simulink model "Dynamic_model_2021b"  (R2021b)
settings: Solver=VariableStepAuto  StartTime=0.0  StopTime=10.0  RelTol=1e-3
values from neighbouring files (symbols this model uses):
  param = struct()    [parameters.m]
libraries: dspmtrx3 x3, sharedtransform x2, matrix_library x1
settings Model: Creator=volko  LastModifiedBy=volko

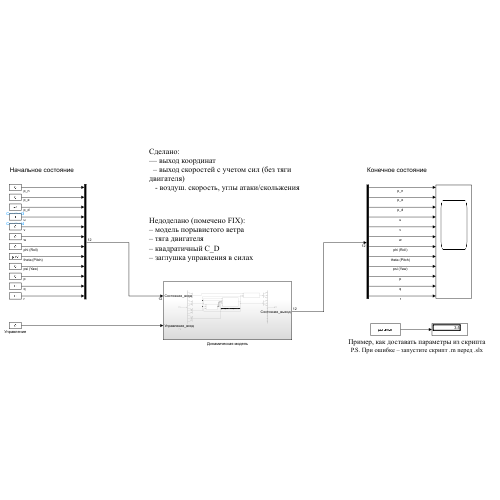
[thumbnail: Simulink's stored preview of the top-level diagram]
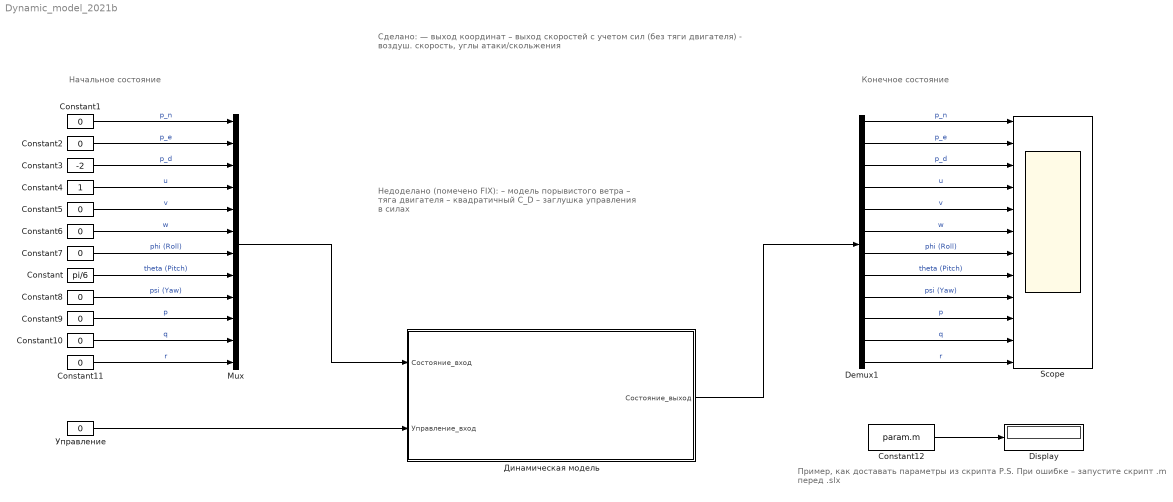
== system Dynamic_model_2021b ==
  note: Сделано:
      | — выход координат
      | – выход скоростей с учетом сил (без тяги двигателя)
      | - воздуш. скорость, углы атаки/скольжения
  note: Пример, как доставать параметры из скрипта
      | P.S. При ошибке – запустите скрипт .m перед .slx
  note: Начальное состояние
  note: Недоделано (помечено FIX):
      | – модель порывистого ветра
      | – тяга двигателя
      | – квадратичный C_D
      | – заглушка управления в силах
  note: Конечное состояние
  Constant : Constant  Value=pi/6
  Constant{1..2,5..11} (9 alike) : Constant  Value=0
  Constant12 : Constant  Value=param.m
  Constant3 : Constant  Value=-2
  Constant4 : Constant
  Demux1 : Demux  Outputs=12
  Display : Display
  Mux : Mux  Inputs=12
  Scope : Scope  NumInputPorts=12
  Динамическая модель : Subsystem
  Управление : Constant  Value=0
  wires:
  Constant7/1 -> Mux/7  "phi (Roll)"
  Demux1/11 -> Scope/11  "q"
  Demux1/1 -> Scope/1  "p_n"
  Mux/1 -> Динамическая модель/1(Состояние_вход)
  Demux1/9 -> Scope/9  "psi (Yaw)"
  Constant2/1 -> Mux/2  "p_e"
  Demux1/3 -> Scope/3  "p_d"
  Constant12/1 -> Display/1
  Demux1/10 -> Scope/10  "p"
  Demux1/12 -> Scope/12  "r"
  Constant10/1 -> Mux/11  "q"
  Управление/1 -> Динамическая модель/2(Управление_вход)
  Demux1/7 -> Scope/7  "phi (Roll)"
  Constant/1 -> Mux/8  "theta (Pitch)"
  Constant3/1 -> Mux/3  "p_d"
  Demux1/5 -> Scope/5  "v"
  Constant5/1 -> Mux/5  "v"
  Demux1/2 -> Scope/2  "p_e"
  Динамическая модель/1(Состояние_выход) -> Demux1/1
  Demux1/6 -> Scope/6  "w"
  Constant11/1 -> Mux/12  "r"
  Constant1/1 -> Mux/1  "p_n"
  Demux1/4 -> Scope/4  "u"
  Constant4/1 -> Mux/4  "u"
  Constant8/1 -> Mux/9  "psi (Yaw)"
  Constant9/1 -> Mux/10  "p"
  Demux1/8 -> Scope/8  "theta (Pitch)"
  Constant6/1 -> Mux/6  "w"

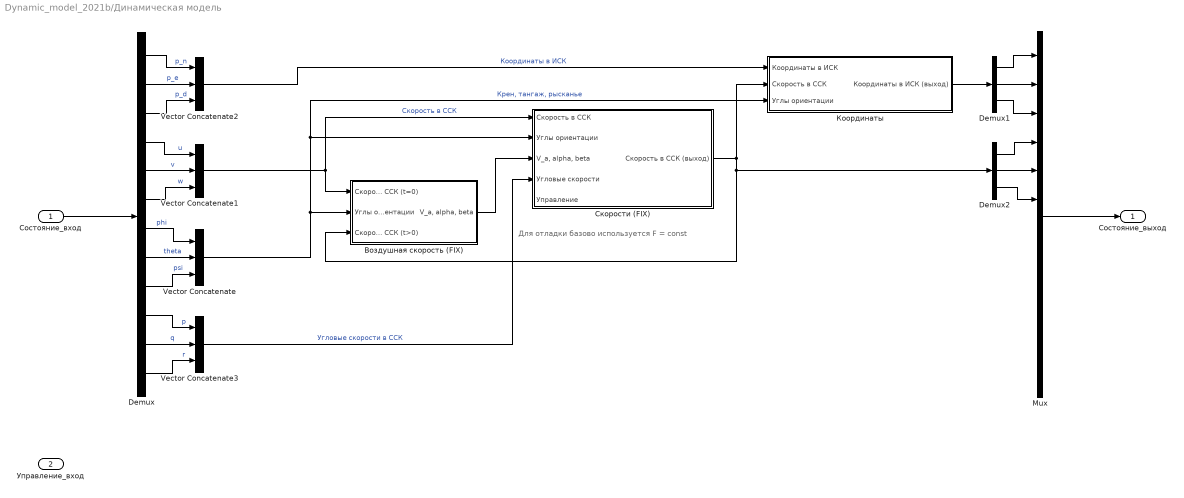
== system Dynamic_model_2021b/Динамическая модель ==
  note: Для отладки базово используется F = const
  Состояние_вход : Inport
  Управление_вход : Inport  Port=2
  Demux : Demux  Outputs=12
  Demux1 : Demux  Outputs=3
  Demux2 : Demux  Outputs=3
  Mux : Mux  Inputs=12
  Vector Concatenate{,1..3} (4 alike) : Concatenate  NumInputs=3
  Воздушная скорость (FIX) : Subsystem
  Координаты : Subsystem
  Скорости (FIX) : Subsystem
  Состояние_выход : Outport
  wires:
  Состояние_вход/1 -> Demux/1
  Demux/1 -> Vector Concatenate2/1  "p_n"
  Demux/2 -> Vector Concatenate2/2  "p_e"
  Demux/3 -> Vector Concatenate2/3  "p_d"
  Demux/4 -> Vector Concatenate1/1  "u"
  Demux/5 -> Vector Concatenate1/2  "v"
  Demux/6 -> Vector Concatenate1/3  "w"
  Demux/7 -> Vector Concatenate/1  "phi"
  Demux/8 -> Vector Concatenate/2  "theta"
  Demux/9 -> Vector Concatenate/3  "psi"
  Demux/10 -> Vector Concatenate3/1  "p"
  Demux/11 -> Vector Concatenate3/2  "q"
  Demux/12 -> Vector Concatenate3/3  "r"
  Vector Concatenate2/1 -> Координаты/1(Координаты в ИСК)  "Координаты в ИСК"
  Vector Concatenate1/1 -> Воздушная скорость (FIX)/1(Скорость в ССК (t=0)), Скорости (FIX)/1(Скорость в ССК)  "Скорость в ССК"
  Vector Concatenate/1 -> Воздушная скорость (FIX)/2(Углы ориентации), Скорости (FIX)/2(Углы ориентации), Координаты/3(Углы ориентации)  "Крен, тангаж, рысканье"
  Координаты/1(Координаты в ИСК (выход)) -> Demux1/1
  Vector Concatenate3/1 -> Скорости (FIX)/4(Угловые скорости)  "Угловые скорости в ССК"
  Mux/1 -> Состояние_выход/1
  Demux1/1 -> Mux/1
  Demux1/2 -> Mux/2
  Demux1/3 -> Mux/3
  Demux2/2 -> Mux/5
  Demux2/1 -> Mux/4
  Demux2/3 -> Mux/6
  Воздушная скорость (FIX)/1("V_a, alpha, beta") -> Скорости (FIX)/3("V_a, alpha, beta")
  Скорости (FIX)/1(Скорость в ССК (выход)) -> Координаты/2(Скорость в ССК), Воздушная скорость (FIX)/3(Скорость в ССК (t>0)), Demux2/1

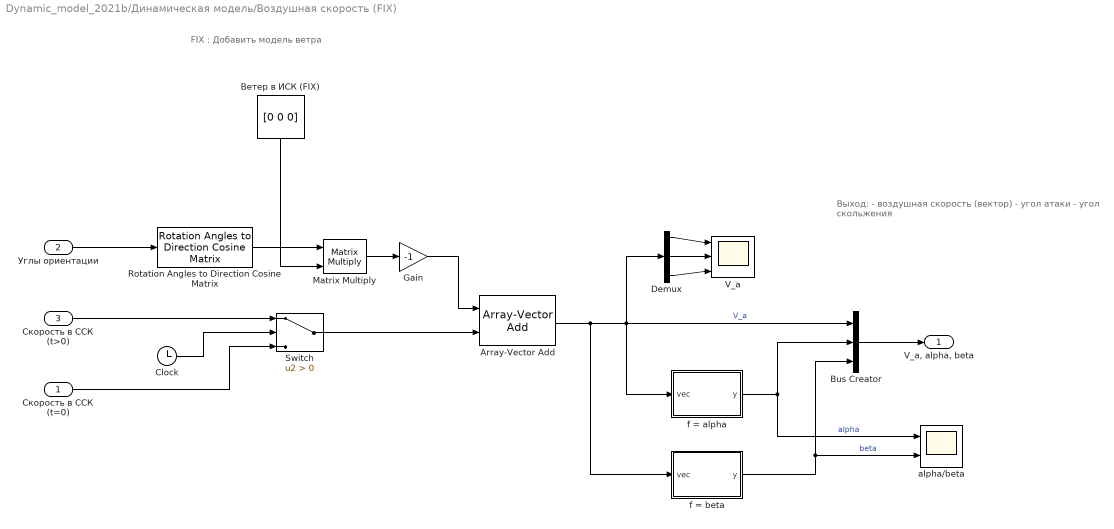
== system Dynamic_model_2021b/Динамическая модель/Воздушная скорость (FIX) ==
  note: Выход:
      | - воздушная скорость (вектор)
      | - угол атаки
      | - угол скольжения
  note: FIX : Добавить модель ветра
  Скорость в ССК (t=0) : Inport
  Углы ориентации : Inport  Port=2
  Скорость в ССК (t>0) : Inport  Port=3
  Array-Vector Add : dspmtrx3/Array-Vector Add  Dimension=1  V_Source=Input port  V_VectFromMask=[0.5 0.25]  prodOutputSignedness=Auto  roundingMode=Floor  overflowMode=off  firstCoeffSignedness=Auto  firstCoeffDataTypeStr=Inherit: Same word length as input  firstCoeffMin=[]  firstCoeffMax=[]  firstCoeffLastDataTypeStr=Inherit: Same word length as input  accumSignedness=Auto  outputSignedness=Auto  outputDataTypeStr=Inherit: Same as accumulator  outputMin=[]  outputMax=[]  outputLastDataTypeStr=Inherit: Same as accumulator
      settings: SourceProductBaseCode=DS
  Bus Creator : BusCreator  Inputs=3
  Clock : Clock
  Demux : Demux  Outputs=3
  Gain : Gain  Gain=-1
  Matrix Multiply : Product  Multiplication=Matrix(*)
  Rotation Angles to Direction Cosine Matrix : sharedtransform/Rotation Angles to Direction Cosine Matrix  rotationOrder=XYZ  aMode=aMode
      settings: SourceProductBaseCode=AE,PW,DR,MT,UV,VE
  Switch : Switch  Criteria=u2 > Threshold
  V_a : Scope  NumInputPorts=3
  alpha/beta : Scope  NumInputPorts=2
  f = alpha : MATLAB Function  TreatAsAtomicUnit=on
  f = beta : MATLAB Function  TreatAsAtomicUnit=on
  Ветер в ИСК (FIX) : Constant  Value=[0 0 0]
  "V_a, alpha, beta" : Outport
  wires:
  Скорость в ССК (t=0)/1 -> Switch/3
  Ветер в ИСК (FIX)/1 -> Matrix Multiply/2
  Array-Vector Add/1 -> Bus Creator/1, Demux/1, f = alpha/1(vec), f = beta/1(vec)  "V_a"
  Rotation Angles to Direction Cosine Matrix/1 -> Matrix Multiply/1
  Углы ориентации/1 -> Rotation Angles to Direction Cosine Matrix/1
  Matrix Multiply/1 -> Gain/1
  f = beta/1(y) -> Bus Creator/3, alpha/beta/2  "beta"
  f = alpha/1(y) -> alpha/beta/1, Bus Creator/2  "alpha"
  Bus Creator/1 -> "V_a, alpha, beta"/1
  Gain/1 -> Array-Vector Add/1
  Demux/1 -> V_a/1
  Demux/2 -> V_a/2
  Demux/3 -> V_a/3
  Clock/1 -> Switch/2
  Скорость в ССК (t>0)/1 -> Switch/1
  Switch/1 -> Array-Vector Add/2

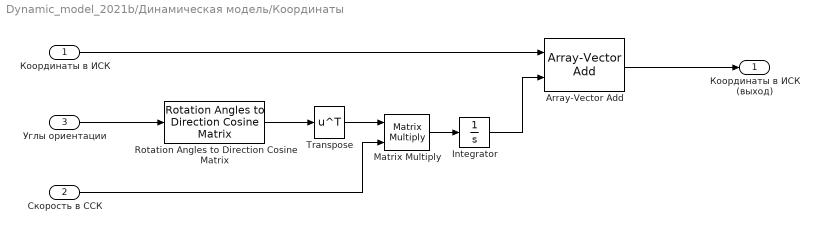
== system Dynamic_model_2021b/Динамическая модель/Координаты ==
  Координаты в ИСК : Inport
  Скорость в ССК : Inport  Port=2
  Углы ориентации : Inport  Port=3
  Array-Vector Add : dspmtrx3/Array-Vector Add  Dimension=1  V_Source=Input port  V_VectFromMask=[0.5 0.25]  prodOutputSignedness=Auto  roundingMode=Floor  overflowMode=off  firstCoeffSignedness=Auto  firstCoeffDataTypeStr=Inherit: Same word length as input  firstCoeffMin=[]  firstCoeffMax=[]  firstCoeffLastDataTypeStr=Inherit: Same word length as input  accumSignedness=Auto  outputSignedness=Auto  outputDataTypeStr=Inherit: Same as accumulator  outputMin=[]  outputMax=[]  outputLastDataTypeStr=Inherit: Same as accumulator
      settings: SourceProductBaseCode=DS
  Integrator : Integrator
  Matrix Multiply : Product  Multiplication=Matrix(*)
  Rotation Angles to Direction Cosine Matrix : sharedtransform/Rotation Angles to Direction Cosine Matrix  rotationOrder=XYZ  aMode=aMode
      settings: SourceProductBaseCode=AE,PW,DR,MT,UV,VE
  Transpose : Math  Operator=transpose  SaturateOnIntegerOverflow=on
  Координаты в ИСК (выход) : Outport
  wires:
  Скорость в ССК/1 -> Matrix Multiply/2
  Integrator/1 -> Array-Vector Add/2
  Rotation Angles to Direction Cosine Matrix/1 -> Transpose/1
  Transpose/1 -> Matrix Multiply/1
  Углы ориентации/1 -> Rotation Angles to Direction Cosine Matrix/1
  Array-Vector Add/1 -> Координаты в ИСК (выход)/1
  Координаты в ИСК/1 -> Array-Vector Add/1
  Matrix Multiply/1 -> Integrator/1

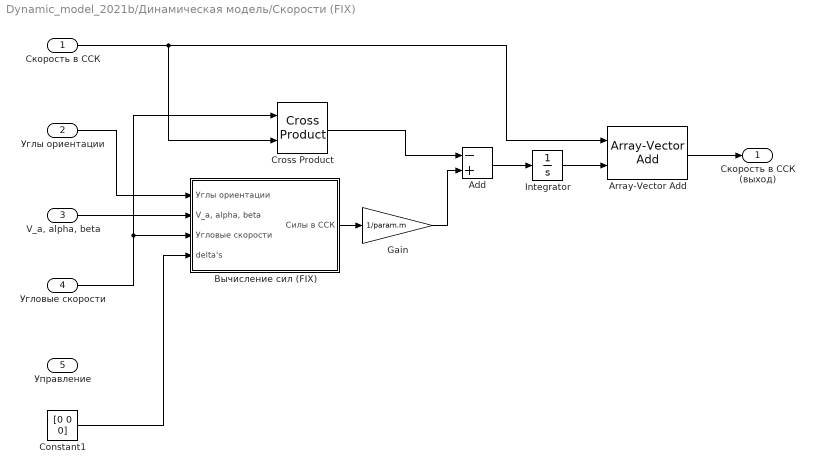
== system Dynamic_model_2021b/Динамическая модель/Скорости (FIX) ==
  Скорость в ССК : Inport
  Углы ориентации : Inport  Port=2
  "V_a, alpha, beta" : Inport  Port=3
  Угловые скорости : Inport  Port=4
  Управление : Inport  Port=5
  Add : Sum  Inputs=-+
  Array-Vector Add : dspmtrx3/Array-Vector Add  Dimension=1  V_Source=Input port  V_VectFromMask=[0.5 0.25]  prodOutputSignedness=Auto  roundingMode=Floor  overflowMode=off  firstCoeffSignedness=Auto  firstCoeffDataTypeStr=Inherit: Same word length as input  firstCoeffMin=[]  firstCoeffMax=[]  firstCoeffLastDataTypeStr=Inherit: Same word length as input  accumSignedness=Auto  outputSignedness=Auto  outputDataTypeStr=Inherit: Same as accumulator  outputMin=[]  outputMax=[]  outputLastDataTypeStr=Inherit: Same as accumulator
      settings: SourceProductBaseCode=DS
  Constant1 : Constant  Value=[0 0 0]
  Cross Product : matrix_library/Cross Product
      settings: SourceProductBaseCode=SL
  Gain : Gain  Gain=1/param.m
  Integrator : Integrator
  Вычисление сил (FIX) : Subsystem
  Скорость в ССК (выход) : Outport
  wires:
  Угловые скорости/1 -> Cross Product/1, Вычисление сил (FIX)/3(Угловые скорости)
  Скорость в ССК/1 -> Array-Vector Add/1, Cross Product/2
  Вычисление сил (FIX)/1(Силы в ССК) -> Gain/1
  Cross Product/1 -> Add/1
  Gain/1 -> Add/2
  Integrator/1 -> Array-Vector Add/2
  Add/1 -> Integrator/1
  Array-Vector Add/1 -> Скорость в ССК (выход)/1
  Углы ориентации/1 -> Вычисление сил (FIX)/1(Углы ориентации)
  "V_a, alpha, beta"/1 -> Вычисление сил (FIX)/2("V_a, alpha, beta")
  Constant1/1 -> Вычисление сил (FIX)/4(delta's)

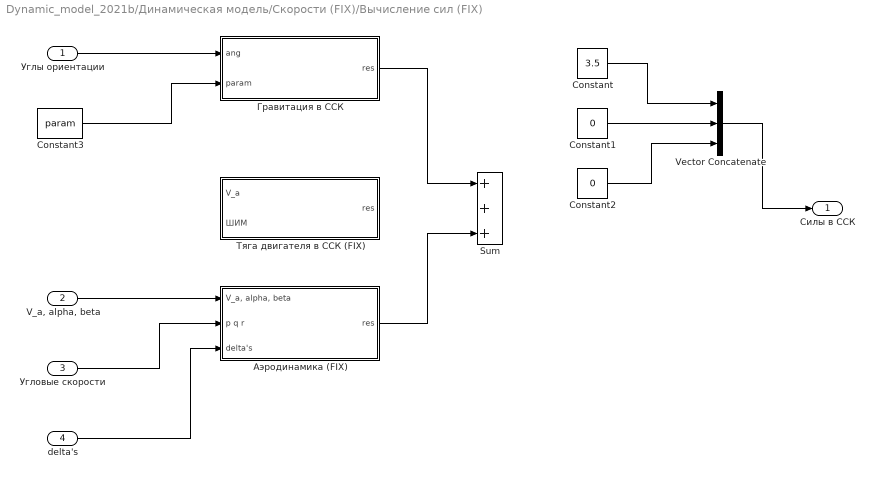
== system Dynamic_model_2021b/Динамическая модель/Скорости (FIX)/Вычисление сил (FIX) ==
  Углы ориентации : Inport
  "V_a, alpha, beta" : Inport  Port=2
  Угловые скорости : Inport  Port=3
  delta's : Inport  Port=4
  Constant : Constant  Value=3.5
  Constant1 : Constant  Value=0
  Constant2 : Constant  Value=0
  Constant3 : Constant  Value=param  OutDataTypeStr=Bus: slBus1
  Sum : Sum  Inputs=+++
  Vector Concatenate : Concatenate  NumInputs=3
  Аэродинамика (FIX) : Subsystem
  Гравитация в ССК : MATLAB Function  TreatAsAtomicUnit=on
  Тяга двигателя в ССК (FIX) : Subsystem
  Силы в ССК : Outport
  wires:
  Constant/1 -> Vector Concatenate/1
  Constant1/1 -> Vector Concatenate/2
  Constant2/1 -> Vector Concatenate/3
  Углы ориентации/1 -> Гравитация в ССК/1(ang)
  Constant3/1 -> Гравитация в ССК/2(param)
  "V_a, alpha, beta"/1 -> Аэродинамика (FIX)/1("V_a, alpha, beta")
  Угловые скорости/1 -> Аэродинамика (FIX)/2(p q r)
  delta's/1 -> Аэродинамика (FIX)/3(delta's)
  Аэродинамика (FIX)/1(res) -> Sum/3
  Гравитация в ССК/1(res) -> Sum/1
  Vector Concatenate/1 -> Силы в ССК/1

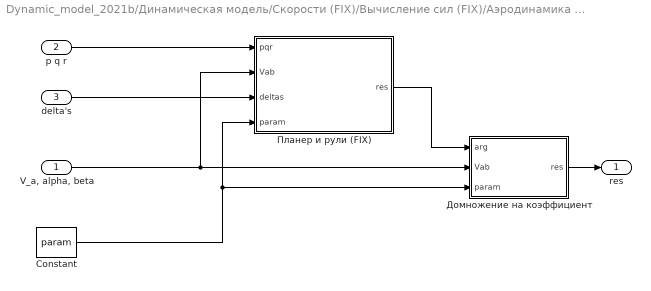
== system Dynamic_model_2021b/Динамическая модель/Скорости (FIX)/Вычисление сил (FIX)/Аэродинамика (FIX) ==
  "V_a, alpha, beta" : Inport
  p q r : Inport  Port=2
  delta's : Inport  Port=3
  Constant : Constant  Value=param  OutDataTypeStr=Bus: slBus1
  Домножение на коэффициент : MATLAB Function  TreatAsAtomicUnit=on
  Планер и рули (FIX) : MATLAB Function  TreatAsAtomicUnit=on
  res : Outport
  wires:
  Домножение на коэффициент/1(res) -> res/1
  Constant/1 -> Планер и рули (FIX)/4(param), Домножение на коэффициент/3(param)
  "V_a, alpha, beta"/1 -> Планер и рули (FIX)/2(Vab), Домножение на коэффициент/2(Vab)
  p q r/1 -> Планер и рули (FIX)/1(pqr)
  Планер и рули (FIX)/1(res) -> Домножение на коэффициент/1(arg)
  delta's/1 -> Планер и рули (FIX)/3(deltas)

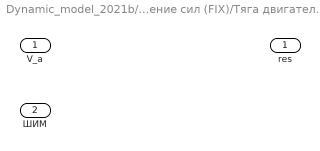
== system Dynamic_model_2021b/Динамическая модель/Скорости (FIX)/Вычисление сил (FIX)/Тяга двигателя в ССК (FIX) ==
  V_a : Inport
  ШИМ : Inport  Port=2
  res : Outport

== matlab function Dynamic_model_2021b/Динамическая модель/Воздушная скорость (FIX)/f = beta ==
  data: vec input; y output
function y = fcn(vec)

y = asin( vec(2) / norm(vec) );

== matlab function Dynamic_model_2021b/Динамическая модель/Воздушная скорость (FIX)/f = alpha ==
  data: vec input; y output
function y = fcn(vec)

y = atan( vec(3) / vec(1) );

== matlab function Dynamic_model_2021b/Динамическая модель/Скорости (FIX)/Вычисление сил (FIX)/Гравитация в ССК ==
  data: ang input; res output; param input
function res = fcn(ang, param)
phi = ang(1);
theta = ang(2);
x = -param.m * param.g * sin(theta);
y = param.m * param.g * cos(theta) * sin(phi);
z = param.m * param.g * cos(theta) * cos(phi);
res = [x y z];

== matlab function Dynamic_model_2021b/Динамическая модель/Скорости (FIX)/Вычисление сил (FIX)/Аэродинамика (FIX)/Домножение на коэффициент ==
  data: arg input; res output; Vab input; param input
function res = fcn(arg, Vab, param)
V_a = Vab(1:3);
res = arg * 0.5 * param.rho * norm(V_a)^2 * param.S;

== matlab function Dynamic_model_2021b/Динамическая модель/Скорости (FIX)/Вычисление сил (FIX)/Аэродинамика (FIX)/Планер и рули (FIX) ==
  data: pqr input; res output; Vab input; deltas input; param input
function res = fcn(pqr, Vab, deltas, param)
% pqr = угловые скорости в ССК
% Vab = воздушная скорость, угол атаки и скольжения
% deltas = отклонения рулей
vV_a = Vab(1:3);
V_a = norm(Vab(1:3));
a = Vab(4);
beta = Vab(5);
p = pqr(1);
q = pqr(2);
r = pqr(3);
delta_a = deltas(1);
delta_e = deltas(2);
delta_r = deltas(3);

%C_D упрощен до линейного !!!!!!!!!!!!!!!!!!!!!!!!!
C_D = param.C_D0 + param.C_Da * a + param.C_Dde * delta_e + param.C_Dq * param.c * q / (2*V_a);
C_L = param.C_L0 + param.C_La * a + param.C_Lde * delta_e + param.C_Lq * param.c * q / (2*V_a);

C = ([cos(a) -sin(a); sin(a) cos(a) ] * [-C_D; -C_L]).';
%C_X = C(1) * sign(vV_a(1));
C_X = C(1);
C_Z = C(2);
C_Y = param.C_Y0 + param.C_Yb * beta + ...
      param.C_Yp * param.b * p / (2*V_a) + param.C_Yr * param.b * r / (2*V_a) +...
      param.C_Yda * delta_a + param.C_Ydr * delta_r;

res = [C_X, C_Y, C_Z];
